simulink model "anfis1"  (R2025b)
settings: Solver=VariableStepAuto  StartTime=0.0  StopTime=20  RelTol=1e-3

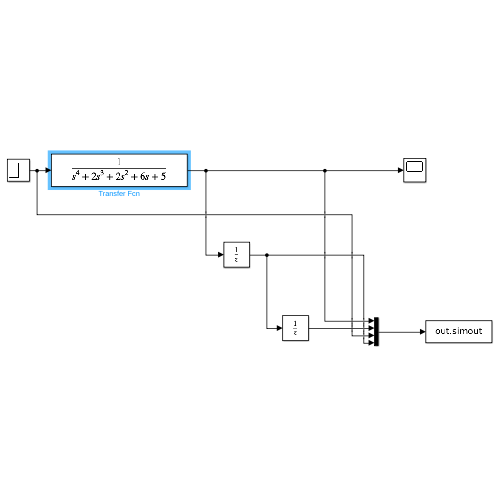
[thumbnail: Simulink's stored preview of the top-level diagram]
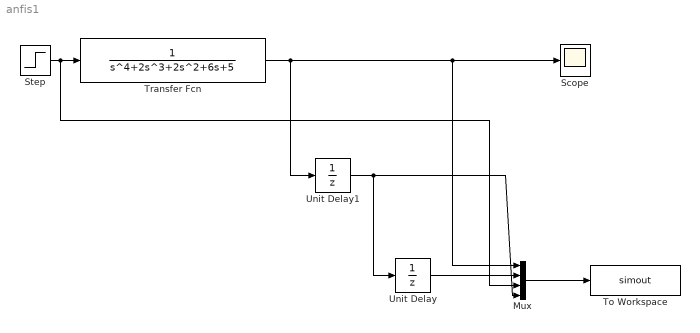
== system anfis1 ==
  Mux : Mux
  Scope : Scope
      settings: ActiveDisplayYMinimum=-0.14537151929163591  ActiveDisplayYMaximum=1.3083436736247234
  Step : Step  SampleTime=0
  To Workspace : ToWorkspace  VariableName=simout  SampleTime=0.1
  Transfer Fcn : TransferFcn  Denominator=[1 2 2 6 5]
  Unit Delay : UnitDelay  SampleTime=-1  HasFrameUpgradeWarning=on
  Unit Delay1 : UnitDelay  SampleTime=-1  HasFrameUpgradeWarning=on
  wires:
  Step/1 -> Transfer Fcn/1, Mux/3
  Transfer Fcn/1 -> Scope/1, Mux/1, Unit Delay1/1
  Unit Delay/1 -> Mux/2
  Unit Delay1/1 -> Unit Delay/1, Mux/4
  Mux/1 -> To Workspace/1
